simulink model "PI_controller"  (R2020a)
settings: Solver=VariableStepAuto  StartTime=0.0  StopTime=120  RelTol=1e-3
values from neighbouring files (symbols this model uses):
  Ki = 30.0    [cruisectrl.sldd]
  Kp = 800.0    [cruisectrl.sldd]
settings Model: DataDictionary=cruisectrl.sldd  Creator=USER  LastModifiedBy=USER
settings DataIOCC: SaveOutput=off  SaveTime=off

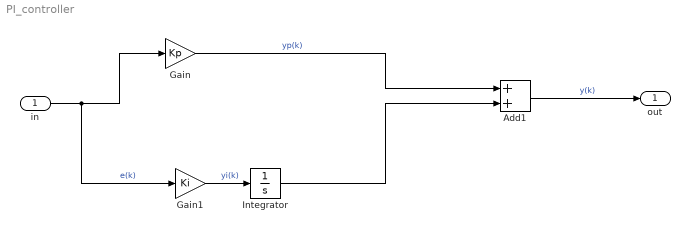
== system PI_controller ==
  in : Inport  OutDataTypeStr=double  PortDimensions=1  SampleTime=0
  Add1 : Sum
  Gain : Gain  Gain=Kp
  Gain1 : Gain  Gain=Ki
  Integrator : Integrator
  out : Outport  OutDataTypeStr=double  PortDimensions=1  SampleTime=0
  wires:
  Add1/1 -> out/1  "y(k)"
  Gain/1 -> Add1/1  "yp(k)"
  in/1 -> Gain/1, Gain1/1  "e(k)"
  Gain1/1 -> Integrator/1  "yi(k)"
  Integrator/1 -> Add1/2
